simulink model "EV_2spd_4AUB10_2023b"  (R2024b)
settings: Solver=VariableStepAuto  StartTime=0.0  StopTime=1800  RelTol=1e-3
values from neighbouring files (symbols this model uses):
  init_SoC = 90    [init_model_opti.m]    (also in run_EV_PT_2spd.m)
  Np = x(4)    [Test_opti.m]    (also in objFun_2spd.m; run_EV_PT_2spd.m)
  Ns = x(5)    [Test_opti.m]    (also in objFun_2spd.m; run_EV_PT_2spd.m)
  Paux = 0    [init_model_opti.m]    (also in run_EV_PT_2spd.m)
  scale_EM = x(3)    [Test_opti.m]    (also in objFun_2spd.m; run_EV_PT_2spd.m)
  T_EM_max = T_EM_max*scale_EM    [run_EV_PT_2spd.m]
undefined symbols (not defined in the file or in its folder): eta_EM_mapG, eta_EM_mapM, theta_EM, w_EM_row, w_EM_upper
libraries: simulink x2, BatteryEstimators x1, DrivingCycle x1, GearSystems x1, GearSystemsControl x1, VehicleBody x1
settings Model: Creator=dadikozyanaa  LastModifiedBy=smaek
settings DebuggingCC: UnconnectedInputMsg=warning  UnconnectedOutputMsg=warning  UnconnectedLineMsg=warning
settings ModelReferenceCC: EnableRefExpFcnMdlSchedulingChecks=on
settings RTWCC: GPUComputeCapability=3.5  DLArmComputeVersion=19.05

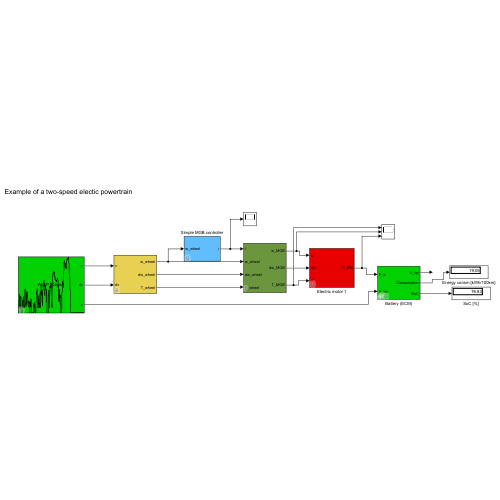
[thumbnail: Simulink's stored preview of the top-level diagram]
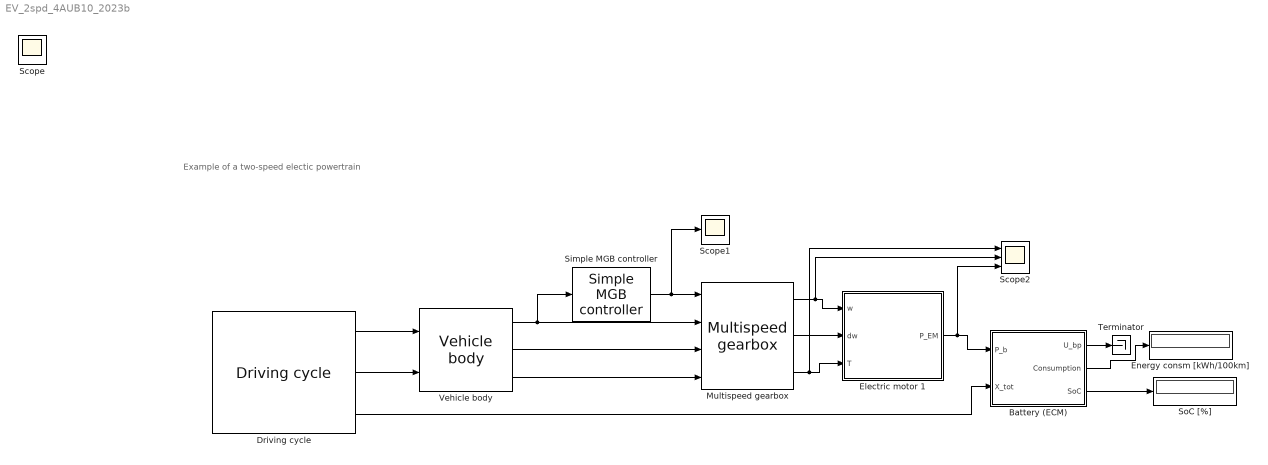
== system EV_2spd_4AUB10_2023b ==
  note: Example of a two-speed electic powertrain
  Battery (ECM) : Subsystem  AncestorBlock=EnergyStorage/Battery (ECM)  InitFcn=% Check if ECMdata already exists in the workspace existingVars = evalin('base', 'who'); if ismember('ECMdata', existingVars) % If ECMdata exists, load it into the mask parameters ECMdata = evalin('base', 'ECMdata'); % Check if values are set, if not set defaults if isempty(get_param(gcb, 'bt_vol')) set_param(gcb, 'bt_vol', num2str(ECMdata.bt_vol)); end if isempty(get_param(gcb, 'bt_cap')) set_param(gcb, 'bt_cap', num2str(ECMdata.bt_cap)); end if isempty(get_param(gcb, 'bt_weight')) set_param(gcb, 'bt_weight', num2str(ECMdata.bt_weight)); end else % If ECMdata doesn't exist, initialize it init_ECM.LoadDataset(gcb); % Call your dataset loading function end  mask(Battery ECM){BattType=High Energy, BattChem=NMC_M35A, init_SoC=init_SoC, bt_Np=Np, bt_Ns=Ns, SoC_low=5, SoC_high=95, U_cell=3.6, Capacity=3.5, CellWeight=50, bt_vol=1022.45, bt_cap=33.67, bt_weight=136.63}
      mask prompts: BattType "<b>Select Battery Type:</b>"; BattChem "<b>Select cell chemistry<\b>"; init_SoC "<b>Initial SoC [%] </b>"; bt_Np "<b>Number of parallel cells [-]</b>"; bt_Ns "<b>Number of cells in series [-]</b>"; SoC_low "<b>Lower SoC boundary [%]</b>"; SoC_high "<b>Upper SoC boundary [%]</b>"; U_cell "<b>Nominal cell Voltage [V]</b>"; Capacity "<b>Nominal cell Capacity [Ah]</b>"; CellWeight "<b>Cell weight [g]</b>"; bt_vol "<b>Battery Pack Voltage [V]</b>"; bt_cap "<b>Battery Pack Capacity [kWh]</b>"; bt_weight "<b>Battery pack Weight [kg]</b>"
      mask help:
      | This block simulates the behaviour of a battery pack by means of a Equivalent Circuit Model (ECM).
      |
      | Battery types & Chemistries:
      | ====
      |           HIgh Power Cells                                        High Energy Cells
      |
      |               - LFP                                                       - NMC
      |               - LTO                                                       - NMC_M35A
      |               - NCA
      |               - NCAVTC
      |
      | Input:
      | =====
      | 	P_BT	Power from/to battery [W]
      | 	x_tot	Total distance [m]
      |
      | Output:
      | =====
      |                            U_b                     Battery pack output voltage [V]
      | 	SoC	Battery state of charge [%]
      | 	cons	Energy consumption [kWh/100km]
      |
      |
      | Please click the help button below for more explanation on the use of this subsystem.
      mask init:
      | % Retrieve mask object
      |     maskObj = Simulink.Mask.get(gcb);
      | 
      |     % Get user-defined parameters from the mask
      |     BattType = get_param(gcb, 'BattType');
      |     BattChem = get_param(gcb, 'BattChem');
      | 
      |     % Determine if input is numerical or string, and convert accordingly
      |     init_SoC = str2double(get_param(gcb, 'init_SoC'));
      |     if isnan(init_SoC)
      |         init_SoC = evalin('base', get_param(gcb, 'init_SoC'));
      |     end
      | 
      |     SoC_low = str2double(get_param(gcb, 'SoC_low'));
      |     if isnan(SoC_low)
      |         SoC_low = evalin('base', get_param(gcb, 'SoC_low'));
      |     end
      |     
      |     SoC_high = str2double(get_param(gcb, 'SoC_high'));
      |     if isnan(SoC_high)
      |         SoC_high = evalin('base', get_param(gcb, 'SoC_high'));
      |     end
      | 
      |     Np = str2double(get_param(gcb, 'bt_Np'));
      |     if isnan(Np)
      |         Np = evalin('base', get_param(gcb, 'bt_Np'));
      |     end
      |     Ns = str2double(get_param(gcb, 'bt_Ns'));
      |     if isnan(Ns)
      |         Ns = evalin('base', get_param(gcb, 'bt_Ns'));
      |     end
      | 
      |     % Define battery cell data directly in mask parameters 
      |     switch BattChem
      |         case 'NMC'
      |             U_cell = 3.7; 
      |             Capacity = 2.6; 
      |             CellWeight = 46.5;
      |             OCV = [3.67137282033677 3.67444281914601 3.68253753930002 3.69462636172811 3.70979566178144 3.72399055404899 3.74044432461285 3.75240892916284 3.76502483557286 3.77943128747097 3.79575092103214 3.81585417119175 3.84109216081761 3.87053450089369 3.90342636561635 3.94227332062956 3.98551629089479 4.03195585445031 4.08406880847627 4.11065689845481 4.13748615299414];
      |             Internal_Resistance = [0.106225776177762 0.102080919410415 0.0982371487638719 0.0917122730547504 0.0847459500877371 0.0806575393392059 0.0775123708858405 0.0755348848509007 0.0741574737127658 0.0732692222665178 0.0729447610492672 0.072936510392724 0.0732980555695696 0.074104227963742 0.0753066920735398 0.0768301415490401 0.078713125536742 0.0790762333647364 0.0735802482063521 0.0723743344246738 0.0695320104391935];
      |             SoC_breakpoints = [0, 0.05, 0.1000, 0.1500, 0.2000, 0.2500, 0.3000, 0.3500, 0.4000, 0.4500, 0.5000, 0.5500, 0.6000, 0.6500, 0.7000, 0.7500, 0.8000, 0.8500, 0.9000, 0.9500, 1.0000];
      |         case 'NMC_M35A'
      |             U_cell = 3.6; 
      |             Capacity = 3.5; 
      |             CellWeight = 50;
      |             OCV = [2.77076488789721 3.08077752214667 3.16461148977458 3.26159785668535 3.35982639556851 3.43918203056113 3.5144454845514 3.55992579373139 3.61574912503331 3.68326088409342 3.74328989315714 3.78941069283519 3.83208501936215 3.86784343598827 3.90493293688704 3.94913484024127 4.01771319883584 4.07048497558508 4.08823629428161 4.08910161280814 4.16271587016724];
      |             Internal_Resistance = [0.0623002821797073 0.0579359998212209 0.0552523962289468 0.0502438642570529 0.0455241026780708 0.0445890100653091 0.0447304630478788 0.0455378869182577 0.0468362388173799 0.0477279263391643 0.0486019764979813 0.0489815180132528 0.0485976128988643 0.0478405730220439 0.0478755262194505 0.0485659942884979 0.0492465105997442 0.0495863122162962 0.0473689399793406 0.0467393658317921 0.044871723483171];
      |             SoC_breakpoints = [0, 0.05, 0.1000, 0.1500, 0.2000, 0.2500, 0.3000, 0.3500, 0.4000, 0.4500, 0.5000, 0.5500, 0.6000, 0.6500, 0.7000, 0.7500, 0.8000, 0.8500, 0.9000, 0.9500, 1.0000];
      |         case 'LFP'
      |             U_cell = 3.3; 
      |             Capacity = 2.56; 
      |             CellWeight = 76;
      |             OCV = [3.03513432281915 3.07250139967424 3.09955393029542 3.14898837202736 3.20077617756473 3.21994889564786 3.23366597676229 3.24376678073082 3.25171275594497 3.25812804369516 3.26246537290231 3.2669068139488 3.27162352983363 3.27745203765021 3.28417677501568 3.29159759804716 3.29895346340881 3.30617668314684 3.33502492162406 3.34329421310162 3.35591224574584];
      |             Internal_Resistance = [0.0249751282445957 0.0226278685626991 0.021191857000342 0.0184416536799028 0.0155902831637008 0.0146514145653925 0.0141848343147171 0.0136710616890657 0.0132470770977912 0.012880372090839 0.0125641465877133 0.0122692618824676 0.0120497113229397 0.0119004364205665 0.0117951282521112 0.0117287804851192 0.011904427055143 0.0119502510938162 0.0104659921279802 0.0101515839817264 0.00965641562577802];
      |             SoC_breakpoints = [0, 0.05, 0.1000, 0.1500, 0.2000, 0.2500, 0.3000, 0.3500, 0.4000, 0.4500, 0.5000, 0.5500, 0.6000, 0.6500, 0.7000, 0.7500, 0.8000, 0.8500, 0.9000, 0.9500, 1.0000];
      |         case 'LTO'
      |             U_cell = 2.9; 
      |             Capacity = 9; 
      |             CellWeight = 270;
      |             OCV = [2.27952244072487 2.28227416698309 2.29092388613957 2.29936558167588 2.30676043310874 2.3196087457949 2.33344555938727 2.34480113096443 2.35401653926263 2.36165796625984 2.36905621514221 2.37426579194657 2.37711763233689 2.38171467477485 2.39306888675058 2.40897873005109 2.43244006987828 2.46077264385788 2.52879853353323 2.55316865849032 2.58412338963041];
      |             Internal_Resistance = [0.00724779322186236 0.0066631133070389 0.00625455281654348 0.0055186455804316 0.00478109281275459 0.00453478056881747 0.00439325805766872 0.00429553553432946 0.0042329015421084 0.00413309226590461 0.00399441831580759 0.00386338638113329 0.00369790587289751 0.00351881833058449 0.00337037197052311 0.00328832711354726 0.00343973637760668 0.00351086661150625 0.00255417405327022 0.00240344190485212 0.00212594418072614];
      |             SoC_breakpoints = [0, 0.05, 0.1000, 0.1500, 0.2000, 0.2500, 0.3000, 0.3500, 0.4000, 0.4500, 0.5000, 0.5500, 0.6000, 0.6500, 0.7000, 0.7500, 0.8000, 0.8500, 0.9000, 0.9500, 1.0000];
      |         case 'NCA'
      |             U_cell = 3.6; 
      |             Capacity = 7.5; 
      |             CellWeight = 320;
      |             OCV = [3.35036548043773 3.44594789198553 3.43606562132141 3.47912366353713 3.51671278530118 3.55040697265237 3.58579878816887 3.61540298047971 3.64744903164519 3.67949211722857 3.71511589625364 3.75222976117785 3.7914764230352 3.83098876463237 3.87002986820703 3.91479374003557 3.96313164617887 4.01628520755549 4.06663105292359 4.11071389878902 4.18791584626149];
      |             Internal_Resistance = [0.0168196717833431 0.0145992308482519 0.0128845965382598 0.0100537729534461 0.00712730867221418 0.00556312319077443 0.00478001722582796 0.00434764693659022 0.004086195925142 0.00390362102173081 0.00378434039674592 0.00369872601029178 0.0036475408987097 0.00364233502941324 0.00368795288814912 0.00378759703264521 0.0039207767368297 0.00406845496394037 0.00410603420474036 0.00415884157880039 0.00417309448362915];
      |             SoC_breakpoints = [0, 0.05, 0.1000, 0.1500, 0.2000, 0.2500, 0.3000, 0.3500, 0.4000, 0.4500, 0.5000, 0.5500, 0.6000, 0.6500, 0.7000, 0.7500, 0.8000, 0.8500, 0.9000, 0.9500, 1.0000];
      |         case 'NCAVTC'
      |             U_cell = 3.7; 
      |             Capacity = 2.1; 
      |             CellWeight = 45;
      |             OCV = [3.47930919380034 3.49679432787047 3.51796392345313 3.55140071966397 3.58819721430289 3.62199422749725 3.64913403670351 3.66898750978676 3.68666912286011 3.70668560228644 3.73255415190538 3.76715408879045 3.80971272306874 3.85914863220091 3.91446075391163 3.97216639301649 4.03099381121653 4.09154695288592 4.15581530120645 4.1874629237389 4.22075558945247];
      |             Internal_Resistance = [0.178279556994958 0.148497003832258 0.129616769381074 0.0947957605294829 0.0603328856923146 0.0561759671943859 0.054873197761985 0.054287790499865 0.0536218436042915 0.0531441319691432 0.0536018523036786 0.0549910993746037 0.0567119827077207 0.0581081393654393 0.0584871393779244 0.0576461827419186 0.0558209698784996 0.048247490631459 0.032503164239043 0.0264746834152617 0.0175369587799402];
      |             SoC_breakpoints = [0, 0.05, 0.1000, 0.1500, 0.2000, 0.2500, 0.3000, 0.3500, 0.4000, 0.4500, 0.5000, 0.5500, 0.6000, 0.6500, 0.7000, 0.7500, 0.8000, 0.8500, 0.9000, 0.9500, 1.0000];
      |         otherwise
      |              U_cell = 0; Capacity = 0; CellWeight = 0;
      |     end
      | 
      |     % Compute total battery pack properties
      |     packVoltage = round(U_cell * Ns,2);
      |     packCapacity = round(Capacity * Np,2);
      |     packWeight = round((CellWeight * Np * Ns)/1000,2);
      | 
      |   
      |     % Set parameters to be directly used inside the subsystem
      |     set_param(gcb, 'U_cell', num2str(U_cell));
      |     set_param(gcb, 'Capacity', num2str(Capacity));
      |     set_param(gcb, 'CellWeight', num2str(CellWeight));
      |     set_param(gcb, 'bt_vol', num2str(packVoltage));
      |     set_param(gcb, 'bt_cap', num2str(packCapacity));
      |     set_param(gcb, 'bt_weight', num2str(packWeight));
      mask Help:
      | <h1>Battery ECM Subsystem Documentation</h1>
      | <h2>Introduction</h2>
      | This block simulates an equivalent circuit model of a battery. It calculates the nominal pack voltage, capacity, and weight based on input parameters such as number of cells in series and parallel.
      | The block accepts P_BT and x_tot as input, which are the power request for the battery and the total distance driven respectively. As outputs, the model gives the battery pack voltage U_b,  State of Charge and energy consumption.
      | 
      | <h3>Battery type and chemistry selection</h3>
      | The first window will give the option to select between two different battery cell types, namely a high energy or a high power cell. Select one of the types by clicking on the corresponding name, whereafter in the second dropdown menu, a cell chemistry needs to be selected. Again, select a chemistry by clicking on the chemistry and clicking APPLY. If the chemistry is correctly selected, the mask should show the correct cell data in the mask.
      | 
      | <h3>Selected cell properties</h3>
      | This container shows the cell properties of the selected cell such as cell voltage, capacity and weight. When selecting a different chemistry, these values are all updated to reflect the selected chemistry. <br>
      | <b> Note: All the cell chemistries in this mask are of the cilindrical type!</b>
      | 
      | <h3>Cell and Pack parameters </h3>
      | The parameters in this container determine size, capacity and operating region of the cells and the entire battery pack. Here, the parameters that can be adjusted are:
      | <ul>
      |     <li><b>Init_SoC</b> : The initial SoC parameter gives a starting point for the battery pack to start simulation. This can be any value between 0% and 100%.</li>
      |     <li><b>Number of parallel strings bt_Np</b>: The total amount of parallel battery strings that are needed in the battery pack, determining the capacity of the pack.</li>
      |     <li><b>Number of cells in series bt_Ns</b> : The total amount of cells in series, determining the total pack voltage.</li>
      |     <li><b>Lower SoC boundary</b> : The lower bound of the battery pack SoC. This can be any value between 10% and 90%.</li>
      |     <li><b>Upper SoC boundary</b> : The upper bound of the battery pack SoC. This can be any value between 10% and 90%.</li>
      | </ul>
      | 
      | The mask is initialized with default values, but all values should be entered manually by hand and applied before the battery pack values change.
      | 
      | <h3>Battery pack specification</h3>
      | In this container, the relevant specifications of the entire battery pack are displayed. The batterypack weight is determined solely based on the amount of cells in the pack, and does not take into account any other structural parts of the batterypack.
      | 
      | <h3>Important Notes</h3>
      | <ul>
      |     <li>When selecting a new chemistry, do not forget to click apply or OK in the mask, otherwise the changes will not take affect!</li>
      |     <li>The values for the battery pack will be updated based on the inputs.</li>
      |     <li>For more information on the used battery cells, please see the extended documentation and datasheets in the data/BT model folder. </li>
      |     <li>The mask accepts workspace variables and numerical values, but only if they are already defined in the model workspace. Otherwise, the model will give an error</li>
      | </ul>
      mask Callback BattType:
      | % Get the selected battery category
      |     cat = get_param(gcb, 'BattType');
      | 
      |     % Determine the chemistry options based on selection
      |     if strcmp(cat, 'High Energy')
      |         newOptions = 'NMC|NMC_M35A';
      |         defaultChem = 'NMC';
      |     elseif strcmp(cat, 'High Power')
      |         newOptions = 'LFP|LTO|NCA|NCAVTC';
      |         defaultChem = 'LFP';
      |     else  % 'None' or any other option
      |         newOptions = 'None';
      |         defaultChem = 'None';
      |     end
      | 
      |     % Access mask object
      |     maskObj = Simulink.Mask.get(gcb);
      | 
      |     % Update the chemistry dropdown
      |     param = maskObj.getParameter('BattChem');
      |     param.TypeOptions = strsplit(newOptions, '|');
      |     param.Value = defaultChem;
      mask TypeOptions BattChem: NMC | NMC_M35A
      mask DialogControl TypeGroup Prompt: BATTERY TYPE AND CHEMISTRY
      mask DialogControl ParameterGroup Prompt: CELL AND PACK PARAMETERS
      mask DialogControl CellProperties Prompt: SELECTED CELL PROPERTIES
      mask DialogControl SpecsGroup Prompt: BATTERY PACK SPECIFICATIONS
  Driving cycle : DrivingCycle/Driving cycle  bool_combine=off  cyclenr=Europe: WLTP Class 3  cyclenr2=Europe: EUDC  gradient_speed=0  cyclerep=1  stepsize=1  autostop=on  slope_bool_cycle=off  mode_bool=off  mode_array=0
      settings: SourceProductName=Driving cycle
  Electric motor 1 : Subsystem  mask(Electric Motor){motortype=Induction (AC), motornumberPM=32 kW, motornumberAC=187 kW, scale_EM=scale_EM, P_aux=Paux, motornumberSim=1}
      mask prompts: motortype "Select electric machine type:"; motornumberPM "Select electric machine model:"; motornumberAC "Select electric machine model:"; scale_EM "Motor scaling factor [-]:"; P_aux "Auxiliary power [W]:"; motornumberSim "Select electric machine number:"
      mask help:
      | This block simulates the behaviour of an electric motor. The block is based on an efficiency map.
      |
      | Input:
      | =====
      | 	w_gear	Speed of the fly wheel [rad/s]
      | 	dw_gear	Acceleration of the fly wheel [rad/s^2]
      | 	T_gear	Torque on the fly wheel [Nm]
      |
      | Output:
      | ======
      | 	P_EM	Power produced by the EM [W]
      mask init:
      | init_EM;
      mask Help: web(which('help_ElectricMotor.html'), '-helpbrowser')
      mask TypeOptions motortype: Permanent Magnet (PMSM) | Induction (AC)
      mask Callback motortype:
      | maskStr = get_param(gcb,'motortype');
      | 
      | switch maskStr
      |     case 'Permanent Magnet (PMSM)'
      |         set_param(gcb,'MaskVisibilities',{'on';'on';'off';'on';'on';'on'}),
      |     case 'Induction (AC)'
      |         set_param(gcb,'MaskVisibilities',{'on';'off';'on';'on';'on';'on'}),
      | end
      mask TypeOptions motornumberPM: 32 kW | 58 kW
      mask TypeOptions motornumberAC: 75 kW | 187 kW
      mask TypeOptions motornumberSim: 1 | 2 | 3 | 4 | 5 | 6 | 7 | 8
      mask DialogControl ParameterGroupVar Prompt: EM type and model
      mask DialogControl Container3 Prompt: Parameters
      mask DialogControl ParameterGroupVar_copy Prompt: EM number
      mask Display:
      | %disp(messageEM, 'texmode', 'on')
      | %plot(w_EM_max, T_EM_max);
  Energy consm [kWh/100km] : Display
  Multispeed gearbox : GearSystems/Multispeed gearbox  Tag=transmission  nr_gears=2  i_1=g1  i_2=g2  i_3=5.378  i_4=3.937  i_5=2.748  i_6=2.748  i_diff=1  e_GT=e_gb  P_GT0=Ploss  w_wheel_min=wem_min
      settings: SourceProductName=Gear systems
  Scope1 : Scope
  Scope2 : Scope  NumInputPorts=3
  Simple MGB controller : GearSystemsControl/Simple MGB controller  nr_gears=2  w_shift2=s1  w_shift3=1e10  w_shift4=1e10  w_shift5=1e10  w_shift6=1e10
      settings: SourceProductName=Gear systems control
  SoC [%] : Display
  Terminator : Terminator
  Vehicle body : VehicleBody/Vehicle body  drivetype=RWD  m_f=mv  mt2m_f=10  A_f=Af  d_wheel=dw  cw=cd  mu=cr
      settings: SourceProductName=Vehicle body
  Scope : Scope
  wires:
  Driving cycle/1 -> Vehicle body/1
  Driving cycle/2 -> Vehicle body/2
  Vehicle body/1 -> Simple MGB controller/1, Multispeed gearbox/2
  Vehicle body/2 -> Multispeed gearbox/3
  Vehicle body/3 -> Multispeed gearbox/4
  Multispeed gearbox/2 -> Electric motor 1/2(dw)
  Multispeed gearbox/3 -> Scope2/1, Electric motor 1/3(T)
  Driving cycle/3 -> Battery (ECM)/2(X_tot)
  Battery (ECM)/3(SoC) -> SoC [%]/1
  Battery (ECM)/2(Consumption) -> Energy consm [kWh/100km]/1
  Multispeed gearbox/1 -> Scope2/2, Electric motor 1/1(w)
  Electric motor 1/1(P_EM) -> Scope2/3, Battery (ECM)/1(P_b)
  Battery (ECM)/1(U_bp) -> Terminator/1
  Simple MGB controller/1 -> Scope1/1, Multispeed gearbox/1

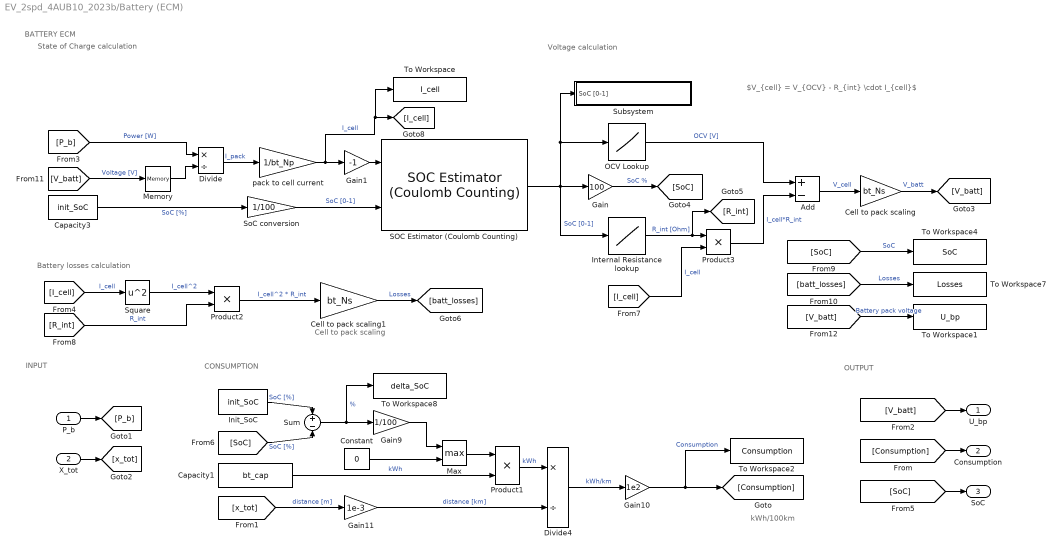
== system EV_2spd_4AUB10_2023b/Battery (ECM) ==
  note: INPUT
  note: CONSUMPTION
  note: OUTPUT
  note: BATTERY ECM
  note: Cell to pack scaling
  note: kWh/100km
  note: Battery losses calculation
  note: State of Charge calculation
  note: Voltage calculation
  note: $V_{cell} = V_{OCV} - R_{int} \cdot I_{cell}$
  P_b : Inport
  X_tot : Inport  Port=2
  Add : Sum  Inputs=+-
  Capacity1 : Constant  Value=bt_cap
  Capacity3 : Constant  Value=init_SoC
  Cell to pack scaling : Gain  Gain=bt_Ns
  Cell to pack scaling1 : Gain  Gain=bt_Ns
  Constant : Constant  Value=0
  Divide : Product  Inputs=*/
  Divide4 : Product  Inputs=*/
  Gain : Gain  Gain=100
  Gain1 : Gain  Gain=-1
  Gain10 : Gain  Gain=1e2
  Gain11 : Gain  Gain=1e-3
  Gain9 : Gain  Gain=1/100
  Init_SoC : Constant  Value=init_SoC
  Internal Resistance lookup : Lookup_n-D  NumberOfTableDimensions=1  BreakpointsForDimension1=SoC_breakpoints  Table=Internal_Resistance  InternalRulePriority=Speed  RndMeth=Simplest
  Max : MinMax  Function=max  Inputs=2
  Memory : Memory  InitialCondition=bt_vol  InheritSampleTime=on  LinearizeAsDelay=on
  OCV Lookup : Lookup_n-D  NumberOfTableDimensions=1  BreakpointsForDimension1=SoC_breakpoints  Table=OCV  InternalRulePriority=Speed  RndMeth=Simplest
  Product1 : Product
  Product2 : Product
  Product3 : Product
  SOC Estimator (Coulomb Counting) : BatteryEstimators/SOC Estimator (Coulomb Counting)  CurrentInputPartition=off  AH=Capacity  Ts=-1
      settings: LibrarySourceBlock=|
      | batt_sl_lib/Estimators/SOC Estimator
      | (Coulomb Counting)
  SoC conversion : Gain  Gain=1/100
  Square : Math  Operator=square
  Subsystem : Subsystem
      mask Display: disp("Battery Full/Empty check")
  Sum : Sum  Inputs=+|-
  To Workspace : ToWorkspace  VariableName=I_cell  SampleTime=-1
  To Workspace1 : ToWorkspace  VariableName=U_bp  SampleTime=-1
  To Workspace2 : ToWorkspace  VariableName=Consumption  SampleTime=-1
  To Workspace4 : ToWorkspace  VariableName=SoC  SampleTime=-1
  To Workspace7 : ToWorkspace  VariableName=Losses  SampleTime=-1
  To Workspace8 : ToWorkspace  VariableName=delta_SoC  SampleTime=-1
  pack to cell current : Gain  Gain=1/bt_Np
  U_bp : Outport
  Consumption : Outport  Port=2
  SoC : Outport  Port=3
  wires:
  [P_b] -> Divide/1  "Power [W]"
  [V_batt] -> To Workspace1/1  "Battery pack voltage"
  [SoC] -> To Workspace4/1  "SoC"
  [batt_losses] -> To Workspace7/1  "Losses"
  Add/1 -> Cell to pack scaling/1  "V_cell"
  Product3/1 -> Add/2  "I_cell*R_int"
  Internal Resistance lookup/1 -> Product3/1, [R_int]  "R_int [Ohm]"
  [I_cell] -> Product3/2  "I_cell"
  SOC Estimator (Coulomb Counting)/1 -> OCV Lookup/1, Subsystem/1(SoC [0-1]), Gain/1, Internal Resistance lookup/1  "SoC [0-1]"
  Gain1/1 -> SOC Estimator (Coulomb Counting)/1
  OCV Lookup/1 -> Add/1  "OCV [V]"
  [R_int] -> Product2/2  "R_int"
  Square/1 -> Product2/1  "I_cell^2"
  [I_cell] -> Square/1  "I_cell"
  Max/1 -> Product1/1
  Gain9/1 -> Max/1
  Constant/1 -> Max/2
  Cell to pack scaling/1 -> [V_batt]  "V_batt"
  Gain/1 -> [SoC]  "SoC %"
  pack to cell current/1 -> [I_cell], To Workspace/1, Gain1/1  "I_cell"
  SoC conversion/1 -> SOC Estimator (Coulomb Counting)/2  "SoC [0-1]"
  Capacity3/1 -> SoC conversion/1  "SoC [%]"
  Divide/1 -> pack to cell current/1  "I_pack"
  Memory/1 -> Divide/2
  [V_batt] -> Memory/1  "Voltage [V]"
  Cell to pack scaling1/1 -> [batt_losses]  "Losses"
  Product2/1 -> Cell to pack scaling1/1  "I_cell^2 * R_int"
  [SoC] -> SoC/1
  [V_batt] -> U_bp/1
  [x_tot] -> Gain11/1  "distance [m]"
  X_tot/1 -> [x_tot]
  P_b/1 -> [P_b]
  [Consumption] -> Consumption/1
  [SoC] -> Sum/2  "SoC [%]"
  Gain11/1 -> Divide4/2  "distance [km]"
  Sum/1 -> Gain9/1, To Workspace8/1  "%"
  Product1/1 -> Divide4/1  "kWh"
  Capacity1/1 -> Product1/2  "kWh"
  Init_SoC/1 -> Sum/1  "SoC [%]"
  Gain10/1 -> [Consumption], To Workspace2/1  "Consumption"
  Divide4/1 -> Gain10/1  "kWh/km"

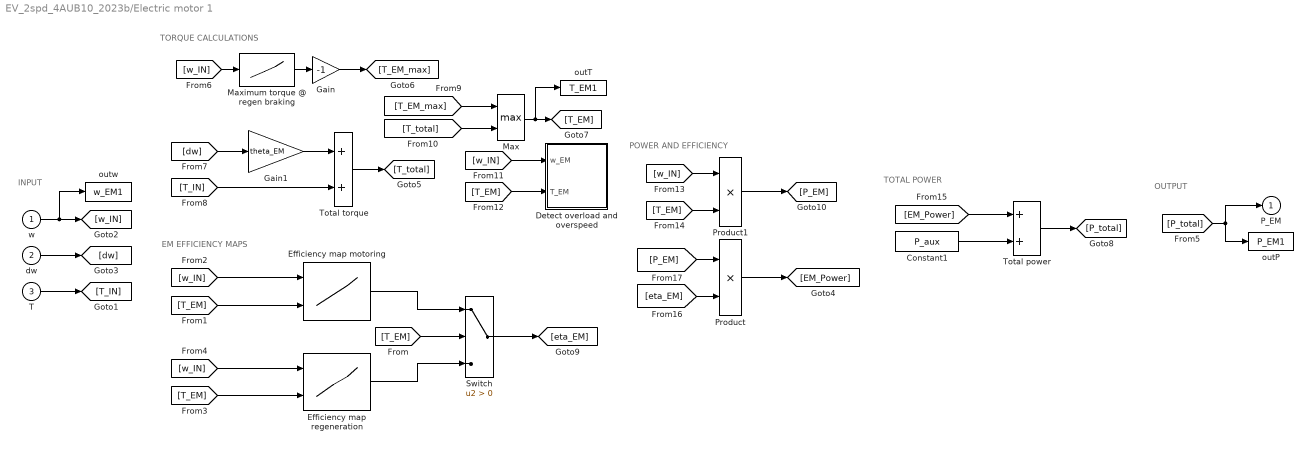
== system EV_2spd_4AUB10_2023b/Electric motor 1 ==
  note: INPUT
  note: TORQUE CALCULATIONS
  note: OUTPUT
  note: EM EFFICIENCY MAPS
  note: POWER AND EFFICIENCY
  note: TOTAL POWER
  w : Inport
  dw : Inport  Port=2
  T : Inport  Port=3
  Constant1 : Constant  Value=P_aux
  Detect overload and overspeed : Subsystem
  Efficiency map motoring : Lookup2D  RowIndex=w_EM_row  ColumnIndex=T_EM_col  Table=eta_EM_mapM  SaturateOnIntegerOverflow=off  InputSameDT=off
  Efficiency map regeneration : Lookup2D  RowIndex=w_EM_row  ColumnIndex=T_EM_col  Table=eta_EM_mapG  SaturateOnIntegerOverflow=off  InputSameDT=off
  Gain : Gain  Gain=-1
  Gain1 : Gain  Gain=theta_EM  SaturateOnIntegerOverflow=on  OutDataTypeStr=Inherit: Same as input  ParamDataTypeStr=Inherit: Same as input
  Max : MinMax  Function=max  Inputs=2
  Maximum torque @ regen braking : Lookup  InputValues=w_EM_row  Table=T_EM_max
  Product : Product  InputSameDT=on  RndMeth=Zero  SaturateOnIntegerOverflow=on  OutDataTypeStr=Inherit: Same as first input
  Product1 : Product
  Switch : Switch  Criteria=u2 > Threshold  SaturateOnIntegerOverflow=off  InputSameDT=off
  Total power : Sum  InputSameDT=on  SaturateOnIntegerOverflow=on  OutDataTypeStr=Inherit: Same as first input
  Total torque : Sum  InputSameDT=on  SaturateOnIntegerOverflow=on  OutDataTypeStr=Inherit: Same as first input
  outP : ToWorkspace  VariableName=P_EM1  SampleTime=-1
  outT : ToWorkspace  VariableName=T_EM1  SampleTime=-1
  outw : ToWorkspace  VariableName=w_EM1  SampleTime=-1
  P_EM : Outport  InitialOutput=0
  wires:
  [P_EM] -> Product/1
  [eta_EM] -> Product/2
  Product1/1 -> [P_EM]
  Switch/1 -> [eta_EM]
  Efficiency map regeneration/1 -> Switch/3
  Efficiency map motoring/1 -> Switch/1
  Total power/1 -> [P_total]
  [EM_Power] -> Total power/1
  Product/1 -> [EM_Power]
  Constant1/1 -> Total power/2
  [T_EM] -> Switch/2
  [w_IN] -> Efficiency map motoring/1
  [T_EM] -> Efficiency map motoring/2
  [T_EM] -> Efficiency map regeneration/2
  [w_IN] -> Efficiency map regeneration/1
  [T_EM] -> Product1/2
  [w_IN] -> Product1/1
  [T_EM] -> Detect overload and overspeed/2(T_EM)
  [w_IN] -> Detect overload and overspeed/1(w_EM)
  Max/1 -> [T_EM], outT/1
  [T_EM_max] -> Max/1
  [T_total] -> Max/2
  Total torque/1 -> [T_total]
  Gain/1 -> [T_EM_max]
  [T_IN] -> Total torque/2
  [dw] -> Gain1/1
  [w_IN] -> Maximum torque @ regen braking/1
  [P_total] -> outP/1, P_EM/1
  w/1 -> [w_IN], outw/1
  dw/1 -> [dw]
  T/1 -> [T_IN]
  Maximum torque @ regen braking/1 -> Gain/1
  Gain1/1 -> Total torque/1

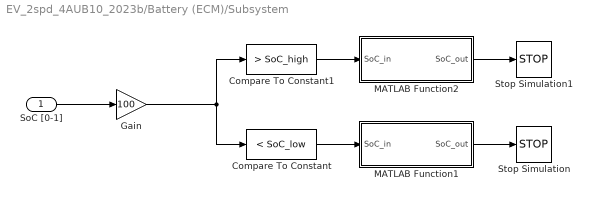
== system EV_2spd_4AUB10_2023b/Battery (ECM)/Subsystem ==
  SoC [0-1] : Inport
  Compare To Constant : simulink/Logic and Bit Operations/Compare To Constant  relop=<  const=SoC_low  OutDataTypeStr=boolean
  Compare To Constant1 : simulink/Logic and Bit Operations/Compare To Constant  relop=>  const=SoC_high  OutDataTypeStr=boolean
  Gain : Gain  Gain=100
  MATLAB Function1 : MATLAB Function  TreatAsAtomicUnit=on
  MATLAB Function2 : MATLAB Function  TreatAsAtomicUnit=on
  Stop Simulation : Stop
  Stop Simulation1 : Stop
  wires:
  Gain/1 -> Compare To Constant/1, Compare To Constant1/1
  SoC [0-1]/1 -> Gain/1
  MATLAB Function1/1(SoC_out) -> Stop Simulation/1
  MATLAB Function2/1(SoC_out) -> Stop Simulation1/1
  Compare To Constant/1 -> MATLAB Function1/1(SoC_in)
  Compare To Constant1/1 -> MATLAB Function2/1(SoC_in)

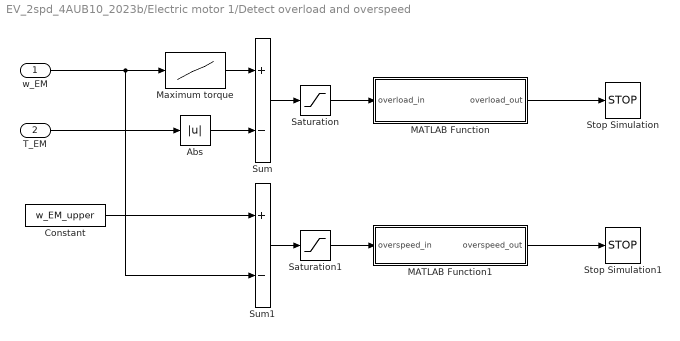
== system EV_2spd_4AUB10_2023b/Electric motor 1/Detect overload and overspeed ==
  w_EM : Inport
  T_EM : Inport  Port=2
  Abs : Abs
  Constant : Constant  Value=w_EM_upper
  MATLAB Function : MATLAB Function  TreatAsAtomicUnit=on
  MATLAB Function1 : MATLAB Function  TreatAsAtomicUnit=on
  Maximum torque : Lookup  InputValues=w_EM_row  Table=T_EM_max
  Saturation : Saturate  UpperLimit=0  LowerLimit=-inf
  Saturation1 : Saturate  UpperLimit=0  LowerLimit=-inf
  Stop Simulation : Stop
  Stop Simulation1 : Stop
  Sum : Sum  Inputs=+-  InputSameDT=on  SaturateOnIntegerOverflow=on  OutDataTypeStr=Inherit: Same as first input
  Sum1 : Sum  Inputs=+-  InputSameDT=on  SaturateOnIntegerOverflow=on  OutDataTypeStr=Inherit: Same as first input
  wires:
  Saturation1/1 -> MATLAB Function1/1(overspeed_in)
  Sum1/1 -> Saturation1/1
  Constant/1 -> Sum1/1
  Saturation/1 -> MATLAB Function/1(overload_in)
  Abs/1 -> Sum/2
  Maximum torque/1 -> Sum/1
  T_EM/1 -> Abs/1
  w_EM/1 -> Sum1/2, Maximum torque/1
  Sum/1 -> Saturation/1
  MATLAB Function/1(overload_out) -> Stop Simulation/1
  MATLAB Function1/1(overspeed_out) -> Stop Simulation1/1

== matlab function EV_2spd_4AUB10_2023b/Electric motor 1/Detect overload and overspeed/MATLAB Function1 ==
  data: overspeed_in input; overspeed_out output
function overspeed_out = overspeed_fnc(overspeed_in)

if overspeed_in~=0
     disp('Simulation stopped due to Motor Overspeed.')
end

overspeed_out = overspeed_in;

== matlab function EV_2spd_4AUB10_2023b/Battery (ECM)/Subsystem/MATLAB Function1 ==
  data: SoC_in input; SoC_out output
function SoC_out = empty(SoC_in)

if SoC_in~=0
    disp('Simulation stopped due to Battery Empty.')
end

SoC_out = SoC_in;

== matlab function EV_2spd_4AUB10_2023b/Battery (ECM)/Subsystem/MATLAB Function2 ==
  data: SoC_in input; SoC_out output
function SoC_out = full(SoC_in)

if SoC_in~=0
    disp('Simulation stopped due to Battery Full.')
end

SoC_out = SoC_in;

== matlab function EV_2spd_4AUB10_2023b/Electric motor 1/Detect overload and overspeed/MATLAB Function ==
  data: overload_in input; overload_out output
function overload_out = overload_fnc(overload_in)

if overload_in~=0
    disp('Simulation stopped due to Motor Overload.')
end

overload_out = overload_in;
